simulink model "AAI"  (R2020a)
settings: Solver=FixedStepAuto  StartTime=0.0  StopTime=10.0  FixedStep=1e-3  RelTol=1e-3  EnableMultiTasking=on
undefined symbols (not defined in the file): D0, D10, D11, D13, D2, D4, D5, D6, D8, PTA0, PTA2, PTB23, PTB9, PTC16, PTC2, PTD0, PTD1, PTD2
libraries: frdmk64flib x11
settings Model: ExtModeTrigDuration=5  Creator=guga  LastModifiedBy=guga
settings OptimizationCC: EnhancedBackFolding=on  PassReuseOutputArgsAs=Individual arguments  ZeroExternalMemoryAtStartup=off  ZeroInternalMemoryAtStartup=off  MaxStackSize=64  OptimizeBlockOrder=speed  DifferentSizesBufferReuse=on  OptimizationCustomize=off  EfficientTunableParamExpr=on
settings DebuggingCC: ParameterTunabilityLossMsg=error
settings HardwareCC: ProdBitPerPointer=32  ProdBitPerSizeT=32  ProdBitPerPtrDiffT=32  ProdLargestAtomicInteger=Long  ProdLargestAtomicFloat=Double  ProdWordSize=32  ProdHWDeviceType=ARM Compatible->ARM Cortex
settings SFSimCC: MATLABDynamicMemAlloc=off
settings RTWCC: SystemTargetFile=ert.tlc  HardwareBoard=NXP FRDM-K64F  TemplateMakefile=ert_default_tmf  Toolchain=GNU Tools for ARM Embedded Processors
settings CodeAppCC: ForceParamTrailComments=on  IgnoreCustomStorageClasses=off  OperatorAnnotations=on  SimulinkDataObjDesc=on  SFDataObjDesc=on  InsertBlockDesc=on

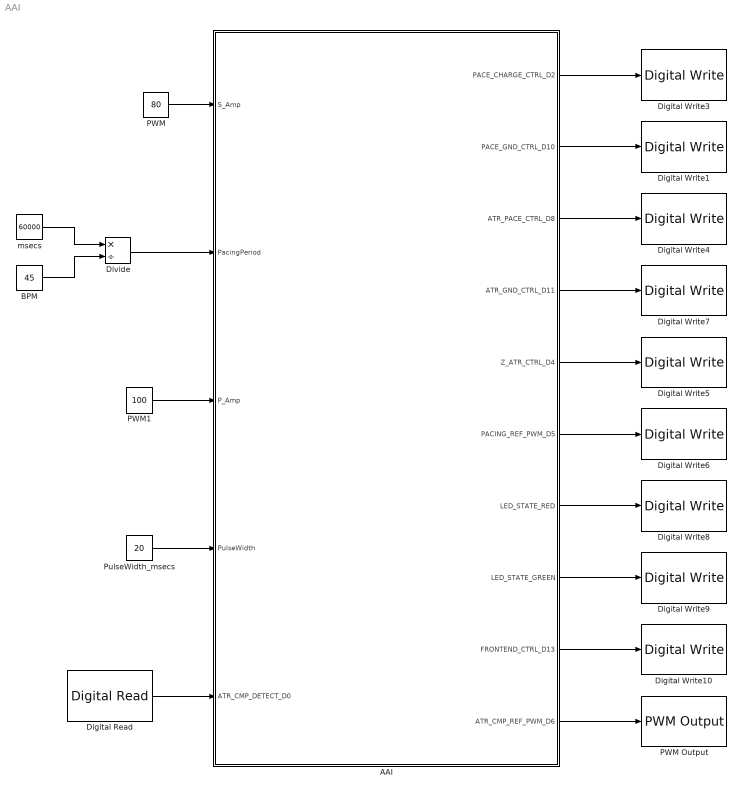
== system AAI ==
  AAI : Stateflow chart  TreatAsAtomicUnit=on
  BPM : Constant  Value=45
  Digital Read : frdmk64flib/Digital Read  Whichpin=PTC16 (D0)  SampleTime=-1
  Digital Write1 : frdmk64flib/Digital Write  Whichpin=PTD0 (D10)
  Digital Write10 : frdmk64flib/Digital Write  Whichpin=PTD1 (D13)
  Digital Write3 : frdmk64flib/Digital Write  Whichpin=PTB9 (D2)
  Digital Write4 : frdmk64flib/Digital Write  Whichpin=PTA0 (D8)
  Digital Write5 : frdmk64flib/Digital Write  Whichpin=PTB23 (D4)
  Digital Write6 : frdmk64flib/Digital Write  Whichpin=PTA2 (D5)
  Digital Write7 : frdmk64flib/Digital Write  Whichpin=PTD2 (D11)
  Digital Write8 : frdmk64flib/Digital Write  Whichpin=RED_LED
  Digital Write9 : frdmk64flib/Digital Write  Whichpin=GREEN_LED
  Divide : Product  Inputs=*/
  PWM : Constant  Value=80
  PWM Output : frdmk64flib/PWM Output  Whichpin=PTC2 (D6)  InitialFrequency=2000  InitialDutyCycle=0
  PWM1 : Constant  Value=100
  PulseWidth_msecs : Constant  Value=20
  msecs : Constant  Value=60000
  wires:
  AAI/4(ATR_GND_CTRL_D11) -> Digital Write7/1
  AAI/8(LED_STATE_GREEN) -> Digital Write9/1
  AAI/5(Z_ATR_CTRL_D4) -> Digital Write5/1
  PWM1/1 -> AAI/3(P_Amp)
  AAI/1(PACE_CHARGE_CTRL_D2) -> Digital Write3/1
  AAI/7(LED_STATE_RED) -> Digital Write8/1
  AAI/3(ATR_PACE_CTRL_D8) -> Digital Write4/1
  AAI/2(PACE_GND_CTRL_D10) -> Digital Write1/1
  AAI/6(PACING_REF_PWM_D5) -> Digital Write6/1
  PWM/1 -> AAI/1(S_Amp)
  AAI/9(FRONTEND_CTRL_D13) -> Digital Write10/1
  AAI/10(ATR_CMP_REF_PWM_D6) -> PWM Output/1
  Digital Read/1 -> AAI/5(ATR_CMP_DETECT_D0)
  ? -> ?
  msecs/1 -> Divide/1
  BPM/1 -> Divide/2
  Divide/1 -> AAI/2(PacingPeriod)
  PulseWidth_msecs/1 -> AAI/4(PulseWidth)

== stateflow chart AAI/AAI ==
  state Pacing
    entry:
    PACING_REF_PWM_D5 = P_Amp;
    PACE_CHARGE_CTRL_D2=0;
    ATR_PACE_CTRL_D8= 1;
    ATR_GND_CTRL_D11= 0;
    PACE_GND_CTRL_D10=1;
    Z_ATR_CTRL_D4=0;
    LED_STATE_RED=false;
    LED_STATE_GREEN=true;
  state Charging_and_Sensing
    entry:
    PACING_REF_PWM_D5 = P_Amp;
    PACE_CHARGE_CTRL_D2=1;
    ATR_PACE_CTRL_D8= 0;
    ATR_GND_CTRL_D11= 1;
    PACE_GND_CTRL_D10=0;
    Z_ATR_CTRL_D4=0;
    LED_STATE_RED=true;
    LED_STATE_GREEN=false;
    FRONTEND_CTRL_D13 = 1;
    ATR_CMP_REF_PWM_D6 = S_Amp;
  (default) -> Charging_and_Sensing
  Pacing -> Charging_and_Sensing : after(PulseWidth,msec)
  Charging_and_Sensing -> (junction 85)
  (junction 85) -> Pacing [order 2] : after(PacingPeriod-PulseWidth,msec)[ATR_CMP_DETECT_D0 == 0]
  (junction 85) -> Charging_and_Sensing [order 1] : [ATR_CMP_DETECT_D0 == 1]
  data: S_Amp input; PacingPeriod input; A_Atrium local; V_Ventricle local; I_Inhibited local; O_None local; VENT_CMP_DETECT_D1 local; VENT_CMP_REF_PWM_D3 local; Z_VENT_CTRL_D7 local; VENT_PACE_CTRL_D9 local; VENT_GND_CTRL_D12 local; GND local; VENT_RECT_SIGNAL_A4_SDA local; ATR_RECT_SIGNAL_A3 local; Z_SIGNAL_A2 local; VENT_SIGNAL_A1 local; ATR_SIGNAL_A0 local; PACE_CHARGE_CTRL_D2 output; PACE_GND_CTRL_D10 output; ATR_PACE_CTRL_D8 output; ATR_GND_CTRL_D11 output; Z_ATR_CTRL_D4 output; PACING_REF_PWM_D5 output; P_Amp input; PulseWidth input; LED_STATE_RED output; LED_STATE_GREEN output; FRONTEND_CTRL_D13 output; ATR_CMP_DETECT_D0 input; ATR_CMP_REF_PWM_D6 output
